simulink model "StateFlow_varB"  (R2022b)
settings: Solver=VariableStepAuto  StartTime=0.0  StopTime=500  FixedStep=0.001  RelTol=1e-3
InitFcn:
  | State_Flow_varB_setting
values from neighbouring files (symbols this model uses):
  Acceptable_press_offset = 5    [State_Flow_varB_setting.m]
  Desired_pressure_in_oxidiser_tank = 40    [State_Flow_varB_setting.m]
  Desired_pressure_in_pressure_section1 = 150    [State_Flow_varB_setting.m]
  Desired_pressure_in_pressure_section2 = 180    [State_Flow_varB_setting.m]
  s = struct    [State_Flow_varB_setting.m]
  Servo_open_limit = 20    [State_Flow_varB_setting.m]
  UDP_FC_send_packet_length = 68    [State_Flow_varB_setting.m]
  UDP_FC_send_sample_time = 0.05    [State_Flow_varB_setting.m]
  UDP_GSE_Curr_loop_receive_sample_time = 0.01    [State_Flow_varB_setting.m]
  UDP_GSE_IO_send_sample_time = 0.05    [State_Flow_varB_setting.m]
  UDP_GSE_send_packet_length = 68    [State_Flow_varB_setting.m]
libraries: simulink x36, slrealtimeiplib x16, slpidlib x6
(part 2 of 3)

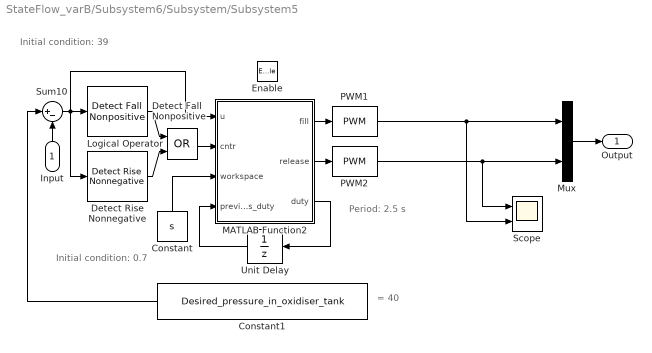
== system StateFlow_varB/Subsystem6/Subsystem/Subsystem5 ==
  note: Initial condition: 39
  note: Period: 2.5 s
  note: Initial condition: 0.7
  note: = 40
  Input : Inport
  Enable : EnablePort  StatesWhenEnabling=reset
  Constant : Constant  Value=s  OutDataTypeStr=Bus: s_bus
  Constant1 : Constant  Value=Desired_pressure_in_oxidiser_tank
  Detect Fall Nonpositive : simulink/Logic and Bit Operations/Detect Fall Nonpositive  vinit=Desired_pressure_in_oxidiser_tank-1  OutDataTypeStr=boolean
  Detect Rise Nonnegative : simulink/Logic and Bit Operations/Detect Rise Nonnegative  vinit=Desired_pressure_in_oxidiser_tank-1  OutDataTypeStr=boolean
  Logical Operator : Logic  Operator=OR  AllPortsSameDT=off  OutDataTypeStr=boolean
  MATLAB Function2 : MATLAB Function  TreatAsAtomicUnit=on
  Mux : Mux  Inputs=2
  PWM1 : simulink/Discontinuities/PWM  DisableCoverage=on  Period=2.5  InitialDelay=0  DisallowZeroDutyCycle=off  RunAtFixedTimeIntervals=off  SampleTime=0.1
  PWM2 : simulink/Discontinuities/PWM  DisableCoverage=on  Period=2.5  InitialDelay=0  DisallowZeroDutyCycle=off  RunAtFixedTimeIntervals=off  SampleTime=0.1
  Scope : Scope  NumInputPorts=2
  Sum10 : Sum  Inputs=|+-
  Unit Delay : UnitDelay  InitialCondition=0.7  SampleTime=-1  HasFrameUpgradeWarning=on
  Output : Outport
  wires:
  Logical Operator/1 -> MATLAB Function2/2(cntr)
  Detect Fall Nonpositive/1 -> Logical Operator/1
  Detect Rise Nonnegative/1 -> Logical Operator/2
  PWM2/1 -> Scope/1, Mux/2
  MATLAB Function2/2(release) -> PWM2/1
  MATLAB Function2/1(fill) -> PWM1/1
  PWM1/1 -> Scope/2, Mux/1
  Unit Delay/1 -> MATLAB Function2/4(previous_duty)
  MATLAB Function2/3(duty) -> Unit Delay/1
  Input/1 -> Sum10/2
  Mux/1 -> Output/1
  Constant/1 -> MATLAB Function2/3(workspace)
  Sum10/1 -> Detect Fall Nonpositive/1, MATLAB Function2/1(u), Detect Rise Nonnegative/1
  Constant1/1 -> Sum10/1

== system StateFlow_varB/Subsystem6/Subsystem/Subsystem6 ==
  Input : Inport
  Enable : EnablePort
  Constant : Constant  Value=Desired_pressure_in_oxidiser_tank
  Dead Zone2 : DeadZone  LowerValue=-Acceptable_press_offset  UpperValue=Acceptable_press_offset
  Gain3 : Gain  Gain=-1
  Mux : Mux  Inputs=2
  Relay3 : Relay  OnSwitchValue=Acceptable_press_offset  OffSwitchValue=0
  Relay4 : Relay  OnSwitchValue=Acceptable_press_offset  OffSwitchValue=0
  Sum7 : Sum  Inputs=|+-
  Output : Outport
  wires:
  Gain3/1 -> Relay4/1
  Relay4/1 -> Mux/2
  Dead Zone2/1 -> Relay3/1, Gain3/1
  Sum7/1 -> Dead Zone2/1
  Relay3/1 -> Mux/1
  Constant/1 -> Sum7/1
  Input/1 -> Sum7/2
  Mux/1 -> Output/1

== system StateFlow_varB/Subsystem6/Subsystem/Subsystem7 ==
  Input : Inport
  Enable : EnablePort
  Constant : Constant  Value=Desired_pressure_in_pressure_section2
  Dead Zone1 : DeadZone  LowerValue=-Acceptable_press_offset  UpperValue=Acceptable_press_offset  SaturateOnIntegerOverflow=off
  Gain2 : Gain  Gain=-1
  Mux : Mux  Inputs=2
  Relay1 : Relay  OnSwitchValue=Acceptable_press_offset  OffSwitchValue=0
  Relay2 : Relay  OnSwitchValue=Acceptable_press_offset  OffSwitchValue=0
  Sum5 : Sum  Inputs=|+-
  Output : Outport
  wires:
  Sum5/1 -> Dead Zone1/1
  Relay1/1 -> Mux/1
  Dead Zone1/1 -> Relay1/1, Gain2/1
  Gain2/1 -> Relay2/1
  Constant/1 -> Sum5/1
  Relay2/1 -> Mux/2
  Input/1 -> Sum5/2
  Mux/1 -> Output/1

== system StateFlow_varB/Subsystem6/Subsystem/Subsystem8 ==
  note: Period: 2 s
  note: Proportional (P): 0.008
  note: Saturation - Upper limit: 1
  note: Saturation - Lower limit: -1
  note: = 180
  Input : Inport
  Enable : EnablePort  StatesWhenEnabling=reset
  Constant : Constant  Value=Desired_pressure_in_pressure_section2
  Gain6 : Gain  Gain=-1
  Mux : Mux  Inputs=2
  PID Controller4 : slpidlib/PID Controller  Controller=P  Form=Parallel  TimeDomain=Discrete-time  UseExternalTs=off  SampleTime=-1  IntegratorMethod=Forward Euler  FilterMethod=Forward Euler  ControllerParametersSource=internal  P=0.008  I=0.01  UseKiTs=off  D=0  N=100  UseFilter=on  TunerSelectOption=Transfer Function Based (PID Tuner App)  InitialConditionSource=internal  InitialConditionForIntegrator=0  InitialConditionForFilter=0  DifferentiatorICPrevScaledInput=0  ExternalReset=none  TrackingMode=off  Kt=1  LimitOutput=on  SatLimitsSource=internal  UpperSaturationLimit=1  LowerSaturationLimit=-1  LinearizeAsGain=on  AntiWindupMode=none  Kb=1  LimitIntegrator=on  UpperIntegratorSaturationLimit=150  LowerIntegratorSaturationLimit=-inf  POutMin=[]  POutMax=[]  IOutMin=[]  IOutMax=[]  DOutMin=[]  DOutMax=[]  NOutMin=[]  NOutMax=[]  SumOutMin=[]  SumOutMax=[]  SaturationOutMin=[]  SaturationOutMax=[]  PParamMin=[]  PParamMax=[]  IParamMin=[]  IParamMax=[]  DParamMin=[]  DParamMax=[]  NParamMin=[]  NParamMax=[]  KbParamMin=[]  KbParamMax=[]  KtParamMin=[]  KtParamMax=[]  KbOutMin=[]  KbOutMax=[]  KtOutMin=[]  KtOutMax=[]  IntegratorOutMin=[]  IntegratorOutMax=[]  FilterOutMin=[]  FilterOutMax=[]  SumI1OutMin=[]  SumI1OutMax=[]  SumI2OutMin=[]  SumI2OutMax=[]  SumI3OutMin=[]  SumI3OutMax=[]  SumI4OutMin=[]  SumI4OutMax=[]  SumDOutMin=[]  SumDOutMax=[]  DifferentiatorOutMin=[]  DifferentiatorOutMax=[]  FilterDiffOutCoefMin=[]  FilterDiffOutCoefMax=[]  ReciprocalOutMin=[]  ReciprocalOutMax=[]  SumDenOutMin=[]  SumDenOutMax=[]  SumNumOutMin=[]  SumNumOutMax=[]  DivideOutMin=[]  DivideOutMax=[]  UdiffTsProdOutMin=[]  UdiffTsProdOutMax=[]  NTsProdOutMin=[]  NTsProdOutMax=[]  UintegralTsProdOutMin=[]  UintegralTsProdOutMax=[]  UngainTsProdOutMin=[]  UngainTsProdOutMax=[]  ClampingZeroOutDataTypeStr=Inherit: Inherit via back propagation  ClampingZeroOutMin=[]  ClampingZeroOutMax=[]  FilterDenConstantOutDataTypeStr=Inherit: Inherit via back propagation  FilterDenConstantOutMin=[]  FilterDenConstantOutMax=[]  PCopyOutDataTypeStr=Inherit: Inherit via back propagation  PCopyOutMin=[]  PCopyOutMax=[]  NCopyOutDataTypeStr=Inherit: Inherit via back propagation  NCopyOutMin=[]  NCopyOutMax=[]  IntegratorContinuousStateAttributes=''  IntegratorStateMustResolveToSignalObject=off  IntegratorRTWStateStorageClass=Auto  FilterContinuousStateAttributes=''  FilterStateMustResolveToSignalObject=off  FilterRTWStateStorageClass=Auto  ParallelPVariant=InternalParameters  IdealPVariant=Disabled  IVariant=Disabled  DVariant=Disabled  IntegratorVariant=Disabled  SatVariant=Enabled  AWVariant=Disabled  PCopyVariant=Disabled  TRVariant=Disabled  FdbkBlocksVariant=Forward  IdealPFdbkVariant=Disabled  SatFdbkVariant=Disabled  DerivativeFilterVariant=Disabled  NVariant=Disabled  NCopyVariant=Disabled_SignalSpec  FilterICVariant=Disabled  IntegratorICVariant=Disabled  ExternalResetVariant=Disabled  TRSumVariant=Passthrough  SumFdbkVariant=Disabled  SumVariant=Passthrough_P  TsampFilterVariant=InternalTs  TsampNgainVariant=Passthrough  TsampIntegralVariant=Disabled_SignalSpec  ExternalSaturationOutDataTypeStr=Inherit: Same as second input
  PWM12 : simulink/Discontinuities/PWM  DisableCoverage=on  Period=2  InitialDelay=0  DisallowZeroDutyCycle=off  RunAtFixedTimeIntervals=off  SampleTime=0.1
  PWM6 : simulink/Discontinuities/PWM  DisableCoverage=on  Period=2  InitialDelay=0  DisallowZeroDutyCycle=off  RunAtFixedTimeIntervals=off  SampleTime=0.1
  Scope : Scope  NumInputPorts=3
  Sum4 : Sum  Inputs=|+-
  Output : Outport
  wires:
  PID Controller4/1 -> PWM6/1, Scope/3, Gain6/1
  Gain6/1 -> PWM12/1
  Mux/1 -> Output/1
  PWM6/1 -> Scope/2, Mux/1
  PWM12/1 -> Scope/1, Mux/2
  Constant/1 -> Sum4/1
  Input/1 -> Sum4/2
  Sum4/1 -> PID Controller4/1

== system StateFlow_varB/Subsystem6/Subsystem/Subsystem9 ==
  note: Initial condition: 149
  note: Period: 2.5 s
  note: Initial condition: 0.2
  note: = 150
  Input : Inport
  Enable : EnablePort  StatesWhenEnabling=reset
  Constant : Constant  Value=s  OutDataTypeStr=Bus: s_bus
  Constant1 : Constant  Value=Desired_pressure_in_pressure_section1
  Detect Fall Nonpositive : simulink/Logic and Bit Operations/Detect Fall Nonpositive  vinit=Desired_pressure_in_pressure_section1-1  OutDataTypeStr=boolean
  Detect Rise Nonnegative : simulink/Logic and Bit Operations/Detect Rise Nonnegative  vinit=Desired_pressure_in_pressure_section1-1  OutDataTypeStr=boolean
  Logical Operator : Logic  Operator=OR  AllPortsSameDT=off  OutDataTypeStr=boolean
  MATLAB Function2 : MATLAB Function  TreatAsAtomicUnit=on
  Mux : Mux  Inputs=2
  PWM1 : simulink/Discontinuities/PWM  DisableCoverage=on  Period=2.5  InitialDelay=0  DisallowZeroDutyCycle=off  RunAtFixedTimeIntervals=off  SampleTime=0.1
  PWM2 : simulink/Discontinuities/PWM  DisableCoverage=on  Period=2.5  InitialDelay=0  DisallowZeroDutyCycle=off  RunAtFixedTimeIntervals=off  SampleTime=0.1
  Scope : Scope  NumInputPorts=2
  Sum10 : Sum  Inputs=|+-
  Unit Delay : UnitDelay  InitialCondition=0.2  SampleTime=-1  HasFrameUpgradeWarning=on
  Output : Outport
  wires:
  Logical Operator/1 -> MATLAB Function2/2(cntr)
  Detect Fall Nonpositive/1 -> Logical Operator/1
  Detect Rise Nonnegative/1 -> Logical Operator/2
  PWM2/1 -> Scope/1, Mux/2
  MATLAB Function2/2(release) -> PWM2/1
  MATLAB Function2/1(fill) -> PWM1/1
  PWM1/1 -> Scope/2, Mux/1
  Unit Delay/1 -> MATLAB Function2/4(previous_duty)
  MATLAB Function2/3(duty) -> Unit Delay/1
  Input/1 -> Sum10/2
  Mux/1 -> Output/1
  Constant/1 -> MATLAB Function2/3(workspace)
  Sum10/1 -> Detect Fall Nonpositive/1, MATLAB Function2/1(u), Detect Rise Nonnegative/1
  Constant1/1 -> Sum10/1

== system StateFlow_varB/Subsystem6/Subsystem3/Subsystem1 ==
  data_prev : Inport
  Constant : Constant  Value=s  OutDataTypeStr=Bus: s_bus
  Display : Display
  Display1 : Display
  MATLAB Function1 : MATLAB Function  TreatAsAtomicUnit=on
  UDP Receive : slrealtimeiplib/UDP Receive  useHostTargetConn=off  ipAddress=UDP_GSE_receive_local_IP  localPort=UDP_GSE_receive_local_PORT  rcvWidth=UDP_GSE_receive_receive_width  rcvFmAny=on  fmAddress='10.10.10.10'  sampleTime=UDP_GSE_Curr_loop_receive_sample_time/4  enableMessage=off  maxPackets=1
  y : Outport
  wires:
  UDP Receive/2 -> Display/1
  data_prev/1 -> MATLAB Function1/2(data_prev)
  MATLAB Function1/1(y) -> y/1
  Constant/1 -> MATLAB Function1/3(workspace)
  UDP Receive/1 -> Display1/1, MATLAB Function1/1(data_new)

== system StateFlow_varB/Subsystem6/Subsystem/Subsystem2/Subsystem1 ==
  Input : Inport
  Enable : EnablePort  StatesWhenEnabling=reset
  Constant : Constant  Value=UDP_GSE_send_packet_length
  Constant2 : Constant  Value=s  OutDataTypeStr=Bus: s_bus
  Constant5 : Constant  Value=s  OutDataTypeStr=Bus: s_bus
  Demux : Demux  Outputs=2
  MATLAB Function : MATLAB Function  TreatAsAtomicUnit=on
  MATLAB Function1 : MATLAB Function  TreatAsAtomicUnit=on
  Scope : Scope
  Scope1 : Scope
  UDP Send : slrealtimeiplib/UDP Send  useHostTargetConn=off  toAddress=UDP_GSE_send_to_IP  toPort=IO_card_2_port  sampleTime=UDP_GSE_IO_send_sample_time  enableMessage=off
  UDP Send1 : slrealtimeiplib/UDP Send  useHostTargetConn=off  toAddress=UDP_GSE_send_to_IP  toPort=IO_card_3_port  sampleTime=UDP_GSE_IO_send_sample_time  enableMessage=off
  wires:
  Input/1 -> Demux/1
  Constant5/1 -> MATLAB Function/2(workspace)
  Demux/1 -> Scope/1, MATLAB Function/1(input)
  Constant2/1 -> MATLAB Function1/2(workspace)
  Demux/2 -> Scope1/1, MATLAB Function1/1(input)
  MATLAB Function/1(code) -> UDP Send/1
  MATLAB Function1/1(code) -> UDP Send1/1
  Constant/1 -> UDP Send/2, UDP Send1/2

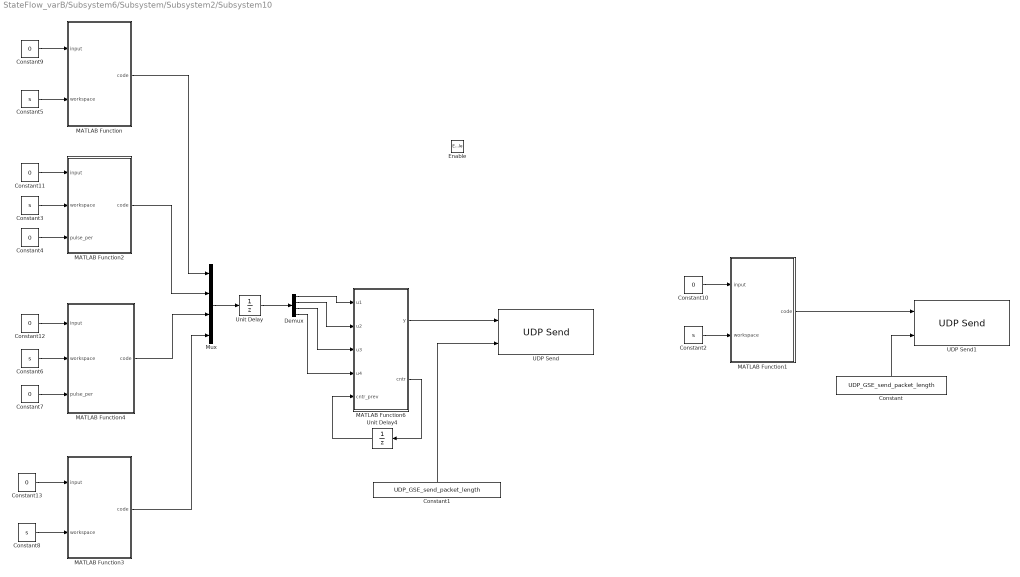
== system StateFlow_varB/Subsystem6/Subsystem/Subsystem2/Subsystem10 ==
  Enable : EnablePort  StatesWhenEnabling=reset
  Constant : Constant  Value=UDP_GSE_send_packet_length
  Constant1 : Constant  Value=UDP_GSE_send_packet_length
  Constant{4,7,9..13} (7 alike) : Constant  Value=0
  Constant{2..3,5..6,8} (5 alike) : Constant  Value=s  OutDataTypeStr=Bus: s_bus
  Demux : Demux
  MATLAB Function : MATLAB Function  TreatAsAtomicUnit=on
  MATLAB Function1 : MATLAB Function  TreatAsAtomicUnit=on
  MATLAB Function2 : MATLAB Function  TreatAsAtomicUnit=on
  MATLAB Function3 : MATLAB Function  TreatAsAtomicUnit=on
  MATLAB Function4 : MATLAB Function  TreatAsAtomicUnit=on
  MATLAB Function6 : MATLAB Function  TreatAsAtomicUnit=on
  Mux : Mux
  UDP Send : slrealtimeiplib/UDP Send  useHostTargetConn=off  toAddress=UDP_GSE_send_to_IP  toPort=IO_card_2_port  sampleTime=UDP_GSE_IO_send_sample_time  enableMessage=off
  UDP Send1 : slrealtimeiplib/UDP Send  useHostTargetConn=off  toAddress=UDP_GSE_send_to_IP  toPort=IO_card_3_port  sampleTime=UDP_GSE_IO_send_sample_time  enableMessage=off
  Unit Delay : UnitDelay  SampleTime=UDP_GSE_IO_send_sample_time*4  HasFrameUpgradeWarning=on
  Unit Delay4 : UnitDelay  InitialCondition=1  SampleTime=UDP_GSE_IO_send_sample_time  HasFrameUpgradeWarning=on
  wires:
  Constant2/1 -> MATLAB Function1/2(workspace)
  MATLAB Function1/1(code) -> UDP Send1/1
  Constant10/1 -> MATLAB Function1/1(input)
  Constant/1 -> UDP Send1/2
  MATLAB Function6/1(y) -> UDP Send/1
  MATLAB Function2/1(code) -> Mux/2
  MATLAB Function4/1(code) -> Mux/3
  MATLAB Function3/1(code) -> Mux/4
  Mux/1 -> Unit Delay/1
  Constant8/1 -> MATLAB Function3/2(workspace)
  Constant12/1 -> MATLAB Function4/1(input)
  Constant6/1 -> MATLAB Function4/2(workspace)
  Constant5/1 -> MATLAB Function/2(workspace)
  Constant4/1 -> MATLAB Function2/3(pulse_per)
  MATLAB Function/1(code) -> Mux/1
  Constant7/1 -> MATLAB Function4/3(pulse_per)
  Constant13/1 -> MATLAB Function3/1(input)
  Constant9/1 -> MATLAB Function/1(input)
  Constant3/1 -> MATLAB Function2/2(workspace)
  Constant11/1 -> MATLAB Function2/1(input)
  Unit Delay/1 -> Demux/1
  Demux/1 -> MATLAB Function6/1(u1)
  Demux/2 -> MATLAB Function6/2(u2)
  Demux/3 -> MATLAB Function6/3(u3)
  Demux/4 -> MATLAB Function6/4(u4)
  MATLAB Function6/2(cntr) -> Unit Delay4/1
  Unit Delay4/1 -> MATLAB Function6/5(cntr_prev)
  Constant1/1 -> UDP Send/2

== system StateFlow_varB/Subsystem6/Subsystem/Subsystem2/Subsystem11 ==
  In1 : Inport
  In2 : Inport  Port=2
  Enable : EnablePort
  UDP Send5 : slrealtimeiplib/UDP Send  useHostTargetConn=off  toAddress=UDP_GSE_send_to_IP  toPort=UDP_GSE_send_to_PORT  sampleTime=UDP_GSE_IO_send_sample_time  enableMessage=off
  wires:
  In2/1 -> UDP Send5/2
  In1/1 -> UDP Send5/1

== system StateFlow_varB/Subsystem6/Subsystem/Subsystem2/Subsystem5 ==
  note: To port: 10003
  note: To IP address: 127.0.0.1
  note: Sample time: 0.05
  note: To port: 10004
  note: To IP address: 127.0.0.1
  note: Sample time: 0.05
  Input : Inport
  Enable : EnablePort  StatesWhenEnabling=reset
  Constant : Constant  Value=UDP_GSE_send_packet_length
  Constant2 : Constant  Value=s  OutDataTypeStr=Bus: s_bus
  Constant5 : Constant  Value=s  OutDataTypeStr=Bus: s_bus
  Demux : Demux  Outputs=2
  MATLAB Function : MATLAB Function  TreatAsAtomicUnit=on
  MATLAB Function1 : MATLAB Function  TreatAsAtomicUnit=on
  UDP Send : slrealtimeiplib/UDP Send  useHostTargetConn=off  toAddress=UDP_GSE_send_to_IP  toPort=IO_card_2_port  sampleTime=UDP_GSE_IO_send_sample_time  enableMessage=off
  UDP Send1 : slrealtimeiplib/UDP Send  useHostTargetConn=off  toAddress=UDP_GSE_send_to_IP  toPort=IO_card_3_port  sampleTime=UDP_GSE_IO_send_sample_time  enableMessage=off
  wires:
  Input/1 -> Demux/1
  Constant5/1 -> MATLAB Function/2(workspace)
  Demux/1 -> MATLAB Function/1(input)
  Constant2/1 -> MATLAB Function1/2(workspace)
  Demux/2 -> MATLAB Function1/1(input)
  MATLAB Function/1(code) -> UDP Send/1
  MATLAB Function1/1(code) -> UDP Send1/1
  Constant/1 -> UDP Send/2, UDP Send1/2

== system StateFlow_varB/Subsystem6/Subsystem/Subsystem2/Subsystem6 ==
  In1 : Inport
  Enable : EnablePort  StatesWhenEnabling=reset
  Constant1 : Constant  Value=UDP_FC_send_packet_length
  Constant3 : Constant  Value=s  OutDataTypeStr=Bus: s_bus
  Constant6 : Constant  Value=s  OutDataTypeStr=Bus: s_bus
  Demux : Demux
  Demux1 : Demux  Outputs=2
  MATLAB Function2 : MATLAB Function  TreatAsAtomicUnit=on
  MATLAB Function4 : MATLAB Function  TreatAsAtomicUnit=on
  MATLAB Function6 : MATLAB Function  TreatAsAtomicUnit=on
  Mux : Mux  Inputs=2
  UDP Send2 : slrealtimeiplib/UDP Send  useHostTargetConn=off  toAddress=UDP_FC_send_to_IP  toPort=IO_card_2_port  sampleTime=UDP_GSE_IO_send_sample_time  enableMessage=off
  Unit Delay2 : UnitDelay  SampleTime=UDP_FC_send_sample_time*2  HasFrameUpgradeWarning=on
  Unit Delay4 : UnitDelay  InitialCondition=1  SampleTime=UDP_FC_send_sample_time  HasFrameUpgradeWarning=on
  wires:
  In1/1 -> Demux/1
  Constant3/1 -> MATLAB Function2/2(workspace)
  Demux/1 -> MATLAB Function2/1(input)
  Constant6/1 -> MATLAB Function4/2(workspace)
  Constant1/1 -> UDP Send2/2
  Demux/4 -> MATLAB Function4/3(pulse_per)
  Demux/2 -> MATLAB Function4/1(input)
  Demux/3 -> MATLAB Function2/3(pulse_per)
  MATLAB Function2/1(code) -> Mux/1
  MATLAB Function4/1(code) -> Mux/2
  Mux/1 -> Unit Delay2/1
  Unit Delay2/1 -> Demux1/1
  MATLAB Function6/2(cntr) -> Unit Delay4/1
  Unit Delay4/1 -> MATLAB Function6/3(cntr_prev)
  Demux1/1 -> MATLAB Function6/1(u1)
  Demux1/2 -> MATLAB Function6/2(u2)
  MATLAB Function6/1(y) -> UDP Send2/1

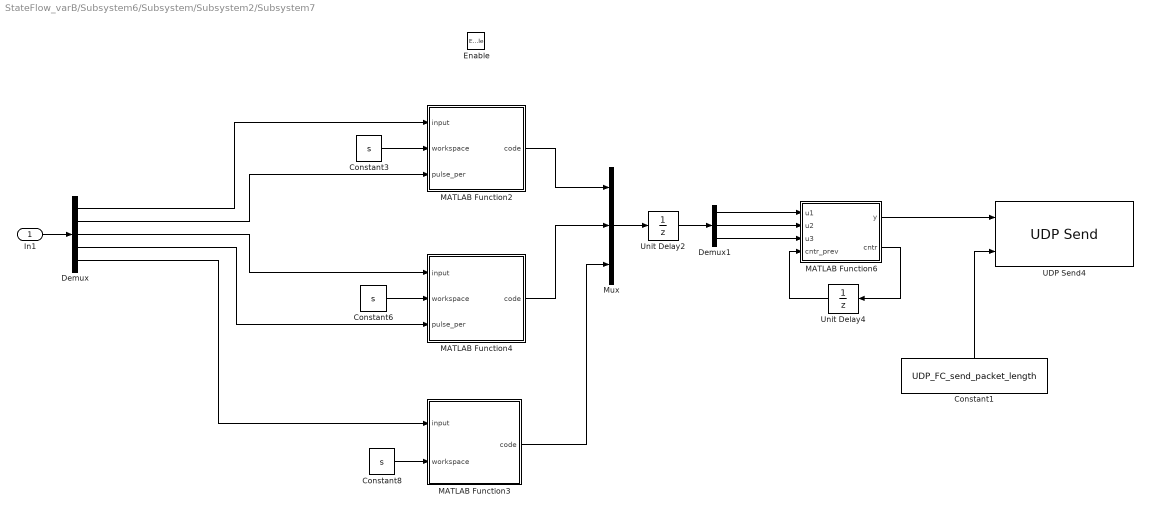
== system StateFlow_varB/Subsystem6/Subsystem/Subsystem2/Subsystem7 ==
  In1 : Inport
  Enable : EnablePort  StatesWhenEnabling=reset
  Constant1 : Constant  Value=UDP_FC_send_packet_length
  Constant3 : Constant  Value=s  OutDataTypeStr=Bus: s_bus
  Constant6 : Constant  Value=s  OutDataTypeStr=Bus: s_bus
  Constant8 : Constant  Value=s  OutDataTypeStr=Bus: s_bus
  Demux : Demux  Outputs=5
  Demux1 : Demux  Outputs=3
  MATLAB Function2 : MATLAB Function  TreatAsAtomicUnit=on
  MATLAB Function3 : MATLAB Function  TreatAsAtomicUnit=on
  MATLAB Function4 : MATLAB Function  TreatAsAtomicUnit=on
  MATLAB Function6 : MATLAB Function  TreatAsAtomicUnit=on
  Mux : Mux  Inputs=3
  UDP Send4 : slrealtimeiplib/UDP Send  useHostTargetConn=off  toAddress=UDP_FC_send_to_IP  toPort=IO_card_2_port  sampleTime=UDP_GSE_IO_send_sample_time  enableMessage=off
  Unit Delay2 : UnitDelay  SampleTime=UDP_GSE_IO_send_sample_time*3  HasFrameUpgradeWarning=on
  Unit Delay4 : UnitDelay  InitialCondition=1  SampleTime=UDP_GSE_IO_send_sample_time  HasFrameUpgradeWarning=on
  wires:
  Constant3/1 -> MATLAB Function2/2(workspace)
  Constant6/1 -> MATLAB Function4/2(workspace)
  Constant1/1 -> UDP Send4/2
  In1/1 -> Demux/1
  Demux/1 -> MATLAB Function2/1(input)
  Demux/4 -> MATLAB Function4/3(pulse_per)
  Demux/2 -> MATLAB Function2/3(pulse_per)
  Demux/3 -> MATLAB Function4/1(input)
  MATLAB Function2/1(code) -> Mux/1
  MATLAB Function4/1(code) -> Mux/2
  Mux/1 -> Unit Delay2/1
  MATLAB Function6/2(cntr) -> Unit Delay4/1
  Demux1/1 -> MATLAB Function6/1(u1)
  Unit Delay4/1 -> MATLAB Function6/4(cntr_prev)
  Demux1/2 -> MATLAB Function6/2(u2)
  Unit Delay2/1 -> Demux1/1
  MATLAB Function6/1(y) -> UDP Send4/1
  Constant8/1 -> MATLAB Function3/2(workspace)
  Demux/5 -> MATLAB Function3/1(input)
  MATLAB Function3/1(code) -> Mux/3
  Demux1/3 -> MATLAB Function6/3(u3)

== system StateFlow_varB/Subsystem6/Subsystem/Subsystem2/Subsystem8 ==
  Input : Inport
  Enable : EnablePort
  Constant : Constant  Value=UDP_GSE_send_packet_length
  Constant8 : Constant  Value=s  OutDataTypeStr=Bus: s_bus
  MATLAB Function3 : MATLAB Function  TreatAsAtomicUnit=on
  UDP Send3 : slrealtimeiplib/UDP Send  useHostTargetConn=off  toAddress=UDP_GSE_send_to_IP  toPort=IO_card_2_port  sampleTime=UDP_GSE_IO_send_sample_time  enableMessage=off
  wires:
  Constant8/1 -> MATLAB Function3/2(workspace)
  Input/1 -> MATLAB Function3/1(input)
  MATLAB Function3/1(code) -> UDP Send3/1
  Constant/1 -> UDP Send3/2

== system StateFlow_varB/Subsystem6/Subsystem/Subsystem2/Subsystem9 ==
  Input : Inport
  Enable : EnablePort  StatesWhenEnabling=reset
  Constant : Constant  Value=UDP_GSE_send_packet_length
  Constant6 : Constant  Value=s  OutDataTypeStr=Bus: s_bus
  Constant8 : Constant  Value=s  OutDataTypeStr=Bus: s_bus
  Demux : Demux  Outputs=3
  Demux1 : Demux  Outputs=2
  MATLAB Function3 : MATLAB Function  TreatAsAtomicUnit=on
  MATLAB Function4 : MATLAB Function  TreatAsAtomicUnit=on
  MATLAB Function6 : MATLAB Function  TreatAsAtomicUnit=on
  Mux : Mux  Inputs=2
  UDP Send4 : slrealtimeiplib/UDP Send  useHostTargetConn=off  toAddress=UDP_FC_send_to_IP  toPort=IO_card_2_port  sampleTime=UDP_GSE_IO_send_sample_time  enableMessage=off
  Unit Delay2 : UnitDelay  SampleTime=UDP_GSE_IO_send_sample_time*2  HasFrameUpgradeWarning=on
  Unit Delay4 : UnitDelay  InitialCondition=1  SampleTime=UDP_GSE_IO_send_sample_time  HasFrameUpgradeWarning=on
  wires:
  Constant6/1 -> MATLAB Function4/2(workspace)
  Constant/1 -> MATLAB Function6/3(length), UDP Send4/2
  Constant8/1 -> MATLAB Function3/2(workspace)
  Demux/1 -> MATLAB Function4/1(input)
  Demux/2 -> MATLAB Function4/3(pulse_per)
  Demux/3 -> MATLAB Function3/1(input)
  Input/1 -> Demux/1
  MATLAB Function4/1(code) -> Mux/1
  MATLAB Function3/1(code) -> Mux/2
  Mux/1 -> Unit Delay2/1
  MATLAB Function6/2(cntr) -> Unit Delay4/1
  Demux1/1 -> MATLAB Function6/1(u1)
  Unit Delay4/1 -> MATLAB Function6/4(cntr_prev)
  Demux1/2 -> MATLAB Function6/2(u2)
  Unit Delay2/1 -> Demux1/1
  MATLAB Function6/1(y) -> UDP Send4/1

== matlab function StateFlow_varB/Subsystem6/Subsystem/Subsystem2/Subsystem1/MATLAB Function ==
  data: input input; code output; workspace input
function code = fcn(input, workspace)

if input == 1
    code = workspace.N2_fill_valve_open; 
else 
    code = workspace.N2_fill_valve_close; 
end
     
end

== matlab function StateFlow_varB/Subsystem6/Subsystem/Subsystem2/Subsystem1/MATLAB Function1 ==
  data: input input; code output; workspace input
function code = fcn(input, workspace)

if input == 1
    code = workspace.N2_release_valve_open;
else
    code = workspace.N2_release_valve_close;
end
     
end

== stateflow chart StateFlow_varB/Subsystem6/Subsystem/Chart ==
  state Pressure_section_pressurization
    entry:
    Pressure_section_pressurization = 1;
    Pressure_section_cntr = 0;
    state Pressure_section_pressurization_Phase_1
      Pressure_section_pressurization_Phase_1 -> (junction 67) [order 1]
      (junction 67) -> (junction 68) [order 1] : [abs(Pressure_section_pressure - Pressure_section_pressure_des) > Acc_Press_Offset]
      (junction 67) -> (junction 69) [order 2]
      (junction 68) -> (junction 70) : {Pressure_section_cntr = 0;}
      (junction 70) -> (junction 69)
      (junction 69) -> (junction 71)
    state Pressure_section_pressurization_Phase_2
      entry:
      Pressure_section_cntr = Pressure_section_cntr + 1
    state Pressure_section_pressurization_Exit_state
      entry:
      Pressure_section_pressurization = 0;
    (default) -> Pressure_section_pressurization_Phase_1
    Pressure_section_pressurization_Phase_1 -> Pressure_section_pressurization_Phase_2 [order 1] : [abs(Pressure_section_pressure - Pressure_section_pressure_des) < Acc_Press_Offset]
    Pressure_section_pressurization_Phase_2 -> Pressure_section_pressurization_Phase_1 [order 2] : [after(Press_Transition_time_const, sec)]
    Pressure_section_pressurization_Phase_2 -> Pressure_section_pressurization_Exit_state [order 1] : [Pressure_section_cntr == Num_dec_time_cycles]
  state Pressure_venting
    entry:
    Pressure_venting = 1;
    Pressure_venting_cntr = 0;
    state Pressure_venting_Phase_1
      Pressure_venting_Phase_1 -> (junction 87) [order 1]
      (junction 87) -> (junction 89) [order 1] : [abs(Oxidiser_tank_pressure - Oxidiser_tank_pressure_des) > Acc_Press_Offset]
      (junction 87) -> (junction 90) [order 2]
      (junction 89) -> (junction 94) : {Pressure_venting_cntr = 0;}
      (junction 94) -> (junction 90)
      (junction 90) -> (junction 92)
    state Pressure_venting_Phase_2
      entry:
      Pressure_venting_cntr = Pressure_venting_cntr + 1;
    state Pressure_venting_Exit_state
      entry:
      Pressure_venting = 0;
    (default) -> Pressure_venting_Phase_1
    Pressure_venting_Phase_1 -> Pressure_venting_Phase_2 [order 1] : [abs(Oxidiser_tank_pressure - Oxidiser_tank_pressure_des) < Acc_Press_Offset]
    Pressure_venting_Phase_2 -> Pressure_venting_Phase_1 [order 2] : [after(Press_Transition_time_const, sec)]
    Pressure_venting_Phase_2 -> Pressure_venting_Exit_state [order 1] : [Pressure_venting_cntr == Num_dec_time_cycles]
  state Oxidiser_fueling_pre_phase
    entry:
    Oxidiser_fueling_pre_phase_cntrl = 1;
    Venting_valve = 0;
    Releasing_valve = 1;
    Oxidiser_fueling_valve = 1;
    state Oxidiser_fueling_pre_phase_init
    state Oxidiser_fueling_exit_state
    (default) -> Oxidiser_fueling_pre_phase_init
    Oxidiser_fueling_pre_phase_init -> Oxidiser_fueling_exit_state : [High_servo_state == 0 && Low_servo_state == 90 && N2O_Fill_valve_state == 0]
  state Oxidiser_fueling
    entry:
    Oxidiser_fueling_cntrl = 1;
    state Oxidiser_fueling_valve_open2
      entry:
      Oxidiser_fueling_valve = 1;
    (default) -> Oxidiser_fueling_valve_open2
  state Oxidiser_fueling_post_phase
    entry:
    Oxidiser_fueling_post_phase_cntrl = 1;
    Oxidiser_fueling_valve = 0;
    Releasing_valve = 0;
    state Oxidiser_fueling_post_phase_init
    state Oxidiser_fueling_post_state
    (default) -> Oxidiser_fueling_post_phase_init
    Oxidiser_fueling_post_phase_init -> Oxidiser_fueling_post_state : [ Low_servo_state == 0 && N2O_Fill_valve_state == 255]
  state Pressure_section_post_pressurization1
    entry:
    Pressure_section_post_pressurization = 1;
    Pressure_section_post_cntr = 0;
    state Pressure_section_post_pressurization_Phase_1
      Pressure_section_post_pressurization_Phase_1 -> (junction 153) [order 1]
      (junction 153) -> (junction 161) [order 1] : [abs(Pressure_section_pressure - Pressure_section_post_pressure_des) > Acc_Press_Offset]
      (junction 153) -> (junction 168) [order 2]
      (junction 161) -> (junction 165) : {Pressure_section_post_cntr = 0;}
      (junction 165) -> (junction 168)
      (junction 168) -> (junction 169)
    state Pressure_section_post_pressurization_Phase_2
      entry:
      Pressure_section_post_cntr = Pressure_section_post_cntr + 1
    state Pressure_section_post_pressurization_Exit_state
      entry:
      Pressure_section_post_pressurization = 0;
    (default) -> Pressure_section_post_pressurization_Phase_1
    Pressure_section_post_pressurization_Phase_2 -> Pressure_section_post_pressurization_Phase_1 [order 2] : [after(Press_Transition_time_const, sec)]
    Pressure_section_post_pressurization_Phase_1 -> Pressure_section_post_pressurization_Phase_2 [order 1] : [abs(Pressure_section_pressure - Pressure_section_post_pressure_des) < Acc_Press_Offset]
    Pressure_section_post_pressurization_Phase_2 -> Pressure_section_post_pressurization_Exit_state [order 1] : [Pressure_section_post_cntr == Num_dec_time_cycles]
  state END_phase
    entry:
    END_Phase_cntrl = 1;
    Releasing_valve = 0;
    Venting_valve = 0;
    Oxidiser_fueling_valve = 0;
  (default) -> Pressure_section_pressurization
  Pressure_section_pressurization_Exit_state -> Pressure_venting : [after(State_transition_time_const,sec)]
  Pressure_venting_Exit_state -> Oxidiser_fueling_pre_phase : [after(State_transition_time_const,sec)]
  Oxidiser_fueling_exit_state -> Oxidiser_fueling : [after(State_transition_time_const,sec)]{Oxidiser_fueling_pre_phase_cntrl = 0;}
  Oxidiser_fueling_valve_open2 -> Oxidiser_fueling_post_phase : [Oxidiser_fueling_valve_time_open == Oxidiser_fueling_exit && Oxidiser_fueling_valve_cntrl_sig == 1 ]{Oxidiser_fueling_cntrl  = 0;}
  Oxidiser_fueling_post_state -> Pressure_section_post_pressurization1 : [after(State_transition_time_const,sec)]{Oxidiser_fueling_post_phase_cntrl = 0;}
  Pressure_section_post_pressurization_Exit_state -> END_phase : [after(State_transition_time_const,sec)]
  data: Pressure_section_pressurization output; Pressure_section_pressure input =150; Pressure_venting output; Oxidiser_fueling_pre_phase_cntrl output; Acc_Press_Offset constant double =Acceptable_press_offset; Press_Transition_time_const constant double =Press_Transition_time_const; Pressure_section_pressure_des constant double =Desired_pressure_in_pressure_section1; Num_dec_time_cycles local =Number_of_decisive_time_cycles; Pressure_venting_cntr local =0; Oxidiser_tank_pressure_des constant double =Desired_pressure_in_oxidiser_tank; Oxidiser_tank_pressure input; State_transition_time_const constant double =Large_State_transition_time_const; Pressure_section_cntr local =0; Venting_valve output; Small_State_transition_time_const local =Small_State_transition_time_const; Oxidiser_fueling_exit constant double =Oxidiser_fueling_exit; Releasing_valve output; Oxidiser_fueling_cntrl output; Oxidiser_fueling_valve output; Oxidiser_fueling_post_phase_cntrl output; Pressure_section_post_cntr local =0; Pressure_section_post_pressure_des constant double =Desired_pressure_in_pressure_section2; END_Phase_cntrl output; Pressure_section_post_pressurization output; N2_Fill_valve_state input; N2_Release_valve_state input; N2O_Fill_valve_state input; N2O_Release_valve_state input; High_servo_state input; Low_servo_state input; Oxidiser_fueling_valve_time_open input; Oxidiser_fueling_valve_cntrl_sig input

== matlab function StateFlow_varB/Subsystem6/Subsystem3/MATLAB Function ==
  data: val_const input; valves_state input; workspace input; u input; y output
function y = fcn(val_const, valves_state, workspace, u)

coder.extrinsic('set_param')

if u >= val_const
    set_param('StateFlow_varB/Subsystem6/Subsystem3/Constant', 'Value', sprintf('%f',u))
    y = 0;
else
   first_valve = valves_state(1);
   second_valve = valves_state(2);
   if ~(first_valve || second_valve)
       if u <= (val_const - workspace.Pressure_drop_const)
           set_param('StateFlow_varB/Subsystem6/Constant', 'Value', '0')
           y = 1;
       else
           y = 0;
       end
   else
       set_param('StateFlow_varB/Subsystem6/Subsystem3/Constant', 'Value', sprintf('%f',u))
       y = 0;
   end
end

end

== matlab function StateFlow_varB/Subsystem6/Subsystem10/MATLAB Function ==
  data: input input; code output; workspace input
function code = fcn(input, workspace)

if input == 1
    code = workspace.N2_fill_valve_open;
else
    code = workspace.N2_fill_valve_close;
end
     
end

== matlab function StateFlow_varB/Subsystem6/Subsystem10/MATLAB Function1 ==
  data: input input; code output; workspace input
function code = fcn(input, workspace)

if input == 1
    code = workspace.N2_release_valve_open;
else
    code = workspace.N2_release_valve_close;
end
     
end

== matlab function StateFlow_varB/Subsystem6/Subsystem10/MATLAB Function2 ==
  data: input input; code output; workspace input; pulse_per input
function code = fcn(input, workspace, pulse_per)

coder.extrinsic('set_param')

if input == 1
    code = workspace.High_servo_open;
else
    code = workspace.High_servo_close;
end


% if pulse_per == 0
%     if input == 1
%         code = workspace.High_servo_open;
%     else
%         code = workspace.High_servo_close;
%     end
% else
%     %comment THIS section if servos are controlled via GSE
%     code = uint8([workspace.FC_ID, workspace.FC_PACKET_LENGTH, workspace.FC_GND_MSG_SERVO_CTRL, workspace.FC_SERVO_PULSE, workspace.FC_SERVO_IGNORE, typecast(uint32(pulse_per), 'uint8'), zeros(1,24)]);
%     set_param('StateFlow_varB/Subsystem6/Constant2', 'Value', '0') %pulse_per is in miliseconds
%     %counting with big endian format
% end

end

== matlab function StateFlow_varB/Subsystem6/Subsystem/Subsystem2/Subsystem5/MATLAB Function ==
  data: input input; code output; workspace input
function code = fcn(input, workspace)

if input == 1
    code = workspace.N2_fill_valve_open; 
else 
    code = workspace.N2_fill_valve_close; 
end
     
end

== matlab function StateFlow_varB/Subsystem6/Subsystem1/MATLAB Function6 ==
  data: u1 input; u2 input; u3 input; u4 input; y output; cntr_prev input; cntr output
function [y, cntr] = fcn(u1, u2, u3, u4, cntr_prev)


y = uint8(zeros(1,68));

switch cntr_prev
    case 1
        y = u1;
    case 2
        y = u2;
    case 3
        y = u3;
    case 4
        y = u4;
end

if cntr_prev < 4
    cntr = cntr_prev + 1;
else
    cntr = 1;
end

== matlab function StateFlow_varB/Subsystem6/Subsystem1/MATLAB Function7 ==
  data: u1 input; u2 input; y output; cntr_prev input; cntr output
function [y, cntr] = fcn(u1, u2, cntr_prev)


y = uint8(zeros(1,68));

switch cntr_prev
    case 1
        y = u1;
    case 2
        y = u2;
end

if cntr_prev < 2
    cntr = cntr_prev + 1;
else
    cntr = 1;
end

== matlab function StateFlow_varB/Subsystem6/Subsystem/Subsystem2/Subsystem5/MATLAB Function1 ==
  data: input input; code output; workspace input
function code = fcn(input, workspace)

if input == 1
    code = workspace.N2_release_valve_open;
else
    code = workspace.N2_release_valve_close;
end
     
end

== matlab function StateFlow_varB/Subsystem6/Subsystem/Subsystem2/Subsystem6/MATLAB Function2 ==
  data: input input; code output; workspace input; pulse_per input
function code = fcn(input, workspace, pulse_per)

coder.extrinsic('set_param')

if input == 1
    code = workspace.High_servo_open;
else
    code = workspace.High_servo_close;
end


% if pulse_per == 0
%     if input == 1
%         code = workspace.High_servo_open;
%     else
%         code = workspace.High_servo_close;
%     end
% else
%     %comment THIS section if servos are controlled via GSE
%     code = uint8([workspace.FC_ID, workspace.FC_PACKET_LENGTH, workspace.FC_GND_MSG_SERVO_CTRL, workspace.FC_SERVO_PULSE, workspace.FC_SERVO_IGNORE, typecast(uint32(pulse_per), 'uint8'), zeros(1,24)]);
%     set_param('StateFlow_varB/Subsystem6/Constant2', 'Value', '0') %pulse_per is in miliseconds
%     %counting with big endian format
% end

end

== matlab function StateFlow_varB/Subsystem6/Subsystem/Subsystem2/Subsystem6/MATLAB Function4 ==
  data: input input; code output; workspace input; pulse_per input
function code = fcn(input, workspace, pulse_per)

coder.extrinsic('set_param')

if input == 1
    code = workspace.Low_servo_open;
else
    code = workspace.Low_servo_close;
end

% if pulse_per == 0
%     if input == 1
%         code = workspace.Low_servo_open;
%     else
%         code = workspace.Low_servo_close;
%     end
% else
%     %comment THIS section if servos are controlled via GSE
%     code = uint8([workspace.FC_ID, workspace.FC_PACKET_LENGTH, workspace.FC_GND_MSG_SERVO_CTRL, workspace.FC_SERVO_PULSE, workspace.FC_SERVO_IGNORE, typecast(uint32(pulse_per), 'uint8'), zeros(1,24)]);
%     set_param('StateFlow_varB/Subsystem6/Constant3', 'Value', '0') %pulse_per is in miliseconds
%     %counting with big endian format
% end

end

== matlab function StateFlow_varB/Subsystem6/Subsystem/Subsystem2/Subsystem7/MATLAB Function2 ==
  data: input input; code output; workspace input; pulse_per input
function code = fcn(input, workspace, pulse_per)

coder.extrinsic('set_param')

if input == 1
    code = workspace.High_servo_open;
else
    code = workspace.High_servo_close;
end

% if pulse_per == 0
%     if input == 1
%         code = workspace.High_servo_open;
%     else
%         code = workspace.High_servo_close;
%     end
% else
%     %comment THIS section if servos are controlled via GSE
%     code = uint8([workspace.FC_ID, workspace.FC_PACKET_LENGTH, workspace.FC_GND_MSG_SERVO_CTRL, workspace.FC_SERVO_PULSE, workspace.FC_SERVO_IGNORE, typecast(uint32(pulse_per), 'uint8'), zeros(1,24)]);
%     set_param('StateFlow_varB/Subsystem6/Constant2', 'Value', '0') %pulse_per is in miliseconds
%     %counting with big endian format
% end

end

== matlab function StateFlow_varB/Subsystem6/Subsystem/Subsystem2/Subsystem7/MATLAB Function4 ==
  data: input input; code output; workspace input; pulse_per input
function code = fcn(input, workspace, pulse_per)

coder.extrinsic('set_param')

if input == 1
    code = workspace.Low_servo_open;
else
    code = workspace.Low_servo_close;
end

% if pulse_per == 0
%     if input == 1
%         code = workspace.Low_servo_open;
%     else
%         code = workspace.Low_servo_close;
%     end
% else
%     %comment THIS section if servos are controlled via GSE
%     code = uint8([workspace.FC_ID, workspace.FC_PACKET_LENGTH, workspace.FC_GND_MSG_SERVO_CTRL, workspace.FC_SERVO_IGNORE, workspace.FC_SERVO_PULSE, typecast(uint32(pulse_per), 'uint8'), zeros(1,24)]);
%     set_param('StateFlow_varB/Subsystem6/Constant3', 'Value', '0') %pulse_per is in miliseconds
%     %counting with big endian format
% end

end

== matlab function StateFlow_varB/Subsystem6/Subsystem/Subsystem2/Subsystem8/MATLAB Function3 ==
  data: input input; code output; workspace input
function code = fcn(input, workspace)

if input == 1
    code = workspace.N2O_fill_valve_open;
else
    code = workspace.N2O_fill_valve_close;
end

end

== matlab function StateFlow_varB/MATLAB Function ==
  data: u input; y output; inside input
function y  = fcn(u, inside)

a = inside.pokus;
y = a;

== matlab function StateFlow_varB/Subsystem6/Subsystem/Subsystem1/MATLAB Function ==
  data: u1 input; y output; u2 input; workspace input
function y = fcn(u1, u2, workspace)

coder.extrinsic('set_param')
set_param('StateFlow_varB/Subsystem6/Constant2', 'Value', u1*workspace.FC_PWM_period) %pulse_per is in miliseconds
set_param('StateFlow_varB/Subsystem6/Constant3', 'Value', u2*workspace.FC_PWM_period) %pulse_per is in miliseconds
%adjust UDP_FC_send_sample_time to larger value (for example 2s)

y = u1;

== matlab function StateFlow_varB/Subsystem6/Subsystem/Subsystem12/MATLAB Function2 ==
  data: u input; fill output; prev_u input; release output; workspace input; duty output; previous_duty input
function [fill, release, duty]= fcn(u, prev_u, workspace, previous_duty)

duty = previous_duty;
if u * prev_u < 0
    duty = previous_duty / 2;
end

if u > 5
    fill = duty;
    release = 0;
elseif u < -5
    release = duty;
    fill = 0;
else
    fill = 0;
    release = 0;
end

== matlab function StateFlow_varB/Subsystem6/Subsystem/Subsystem16/MATLAB Function2 ==
  data: u input; cntr input; fill output; release output; workspace input; duty output; previous_duty input
function [fill, release, duty]= fcn(u, ...
                                    cntr, ...
                                    workspace, ...
                                    previous_duty)

%Halving duty cycle
duty = previous_duty;
if cntr
    duty = previous_duty / 2;
end

%Deciding which valve should be open
if u > 5
    fill = duty;
    release = 0;
elseif u < -5
    release = duty;
    fill = 0;
else
    fill = 0;
    release = 0;
end

== matlab function StateFlow_varB/Subsystem6/Subsystem/Subsystem5/MATLAB Function2 ==
  data: u input; cntr input; fill output; release output; workspace input; duty output; previous_duty input
function [fill, release, duty]= fcn(u, ...
                                    cntr, ...
                                    workspace, ...
                                    previous_duty)

%Halving duty cycle
duty = previous_duty;
if cntr
    duty = previous_duty / 2;
end

%Deciding which valve should be open
if u > workspace.Acceptable_press_offset
    fill = duty;
    release = 0;
elseif u < -workspace.Acceptable_press_offset
    release = duty;
    fill = 0;
else
    fill = 0;
    release = 0;
end

== matlab function StateFlow_varB/Subsystem6/Subsystem/Subsystem14/MATLAB Function ==
  data: u1 input; y output; u2 input; workspace input
function y = fcn(u1, u2, workspace)

coder.extrinsic('set_param')
set_param('StateFlow_varB/Subsystem6/Constant2', 'Value', u1*workspace.FC_PWM_period) %pulse_per is in miliseconds
set_param('StateFlow_varB/Subsystem6/Constant3', 'Value', u2*workspace.FC_PWM_period) %pulse_per is in miliseconds
%adjust UDP_FC_send_sample_time to larger value (for example 2s)

y = u1;

== matlab function StateFlow_varB/Subsystem6/Subsystem/Subsystem2/Subsystem9/MATLAB Function4 ==
  data: input input; code output; workspace input; pulse_per input
function code = fcn(input, workspace, pulse_per)

coder.extrinsic('set_param')

if input == 1
    code = workspace.Low_servo_open;
else
    code = workspace.Low_servo_close;
end


% if pulse_per == 0
%     if input == 1
%         code = workspace.Low_servo_open;
%     else
%         code = workspace.Low_servo_close;
%     end
% else
%     %comment THIS section if servos are controlled via GSE
%     code = uint8([workspace.FC_ID, workspace.FC_PACKET_LENGTH, workspace.FC_GND_MSG_SERVO_CTRL, workspace.FC_SERVO_IGNORE, workspace.FC_SERVO_PULSE, typecast(uint32(pulse_per), 'uint8'), zeros(1,24)]);
%     set_param('StateFlow_varB/Subsystem6/Constant3', 'Value', '0') %pulse_per is in miliseconds
%     %counting with big endian format
% end

end

== matlab function StateFlow_varB/Subsystem6/Subsystem/Subsystem2/Subsystem9/MATLAB Function3 ==
  data: input input; code output; workspace input
function code = fcn(input, workspace)

if input == 1
    code = workspace.N2O_fill_valve_open;
else
    code = workspace.N2O_fill_valve_close;
end

end

== matlab function StateFlow_varB/Subsystem6/Subsystem/Subsystem2/Subsystem10/MATLAB Function ==
  data: input input; code output; workspace input
function code = fcn(input, workspace)

if input == 1
    code = workspace.N2_fill_valve_open; 
else 
    code = workspace.N2_fill_valve_close; 
end
     
end

== matlab function StateFlow_varB/Subsystem6/Subsystem/Subsystem2/Subsystem10/MATLAB Function1 ==
  data: input input; code output; workspace input
function code = fcn(input, workspace)

if input == 1
    code = workspace.N2_release_valve_open;
else
    code = workspace.N2_release_valve_close;
end
     
end

== matlab function StateFlow_varB/Subsystem6/Subsystem/Subsystem2/Subsystem10/MATLAB Function2 ==
  data: input input; code output; workspace input; pulse_per input
function code = fcn(input, workspace, pulse_per)

coder.extrinsic('set_param')

if input == 1
    code = workspace.High_servo_open;
else
    code = workspace.High_servo_close;
end


% if pulse_per == 0
%     if input == 1
%         code = workspace.High_servo_open;
%     else
%         code = workspace.High_servo_close;
%     end
% else
%     comment THIS section if servos are controlled via GSE
%     code = uint8([workspace.FC_ID, workspace.FC_PACKET_LENGTH, workspace.FC_GND_MSG_SERVO_CTRL, workspace.FC_SERVO_PULSE, workspace.FC_SERVO_IGNORE, typecast(uint32(pulse_per), 'uint8'), zeros(1,24)]);
%     set_param('StateFlow_varB/Subsystem6/Constant2', 'Value', '0') %pulse_per is in miliseconds
%     counting with big endian format
% end

end

== matlab function StateFlow_varB/Subsystem6/Subsystem/Subsystem2/Subsystem10/MATLAB Function3 ==
  data: input input; code output; workspace input
function code = fcn(input, workspace)

if input == 1
    code = workspace.N2O_fill_valve_open;
else
    code = workspace.N2O_fill_valve_close;
end

end

== matlab function StateFlow_varB/Subsystem6/Subsystem/Subsystem2/Subsystem10/MATLAB Function4 ==
  data: input input; code output; workspace input; pulse_per input
function code = fcn(input, workspace, pulse_per)

coder.extrinsic('set_param')

if input == 1
    code = workspace.Low_servo_open;
else
    code = workspace.Low_servo_close;
end


% if pulse_per == 0
%     if input == 1
%         code = workspace.Low_servo_open;
%     else
%         code = workspace.Low_servo_close;
%     end
% else
%     %comment THIS section if servos are controlled via GSE
%     code = uint8([workspace.FC_ID, workspace.FC_PACKET_LENGTH, workspace.FC_GND_MSG_SERVO_CTRL, workspace.FC_SERVO_IGNORE, workspace.FC_SERVO_PULSE, typecast(uint32(pulse_per), 'uint8'), zeros(1,24)]);
%     set_param('StateFlow_varB/Subsystem6/Constant3', 'Value', '0') %pulse_per is in miliseconds
%     %counting with big endian format
% end

end

== matlab function StateFlow_varB/Subsystem6/Subsystem10/MATLAB Function3 ==
  data: input input; code output; workspace input
function code = fcn(input, workspace)

if input == 1
    code = workspace.N2O_fill_valve_open;
else
    code = workspace.N2O_fill_valve_close;
end

end

== matlab function StateFlow_varB/Subsystem6/Subsystem10/MATLAB Function4 ==
  data: input input; code output; workspace input; pulse_per input
function code = fcn(input, workspace, pulse_per)

coder.extrinsic('set_param')

if input == 1
    code = workspace.Low_servo_open;
else
    code = workspace.Low_servo_close;
end


% if pulse_per == 0
%     if input == 1
%         code = workspace.Low_servo_open;
%     else
%         code = workspace.Low_servo_close;
%     end
% else
%     comment THIS section if servos are controlled via GSE
%     code = uint8([workspace.FC_ID, workspace.FC_PACKET_LENGTH, workspace.FC_GND_MSG_SERVO_CTRL, workspace.FC_SERVO_IGNORE, workspace.FC_SERVO_PULSE, typecast(uint32(pulse_per), 'uint8'), zeros(1,24)]);
%     set_param('StateFlow_varB/Subsystem6/Constant3', 'Value', '0') %pulse_per is in miliseconds
%     counting with big endian format
% end

end

== matlab function StateFlow_varB/Subsystem6/Subsystem10/MATLAB Function5 ==
  data: input input; code output; workspace input
function code = fcn(input, workspace)

if input == 1
    code = workspace.N2O_release_valve_open;
else
    code = workspace.N2O_release_valve_close;
end

end

== matlab function StateFlow_varB/Subsystem6/Subsystem1/MATLAB Function ==
  data: input input; code output; workspace input
function code = fcn(input, workspace)

if input == 1
    code = workspace.N2_fill_valve_open; 
else 
    code = workspace.N2_fill_valve_close; 
end
     
end

== matlab function StateFlow_varB/Subsystem6/Subsystem1/MATLAB Function1 ==
  data: input input; code output; workspace input
function code = fcn(input, workspace)

if input == 1
    code = workspace.N2_release_valve_open;
else
    code = workspace.N2_release_valve_close;
end
     
end

== matlab function StateFlow_varB/Subsystem6/Subsystem1/MATLAB Function2 ==
  data: input input; code output; workspace input; pulse_per input
function code = fcn(input, workspace, pulse_per)

coder.extrinsic('set_param')

if input == 1
    code = workspace.High_servo_open;
else
    code = workspace.High_servo_close;
end


% if pulse_per == 0
%     if input == 1
%         code = workspace.High_servo_open;
%     else
%         code = workspace.High_servo_close;
%     end
% else
%     comment THIS section if servos are controlled via GSE
%     code = uint8([workspace.FC_ID, workspace.FC_PACKET_LENGTH, workspace.FC_GND_MSG_SERVO_CTRL, workspace.FC_SERVO_PULSE, workspace.FC_SERVO_IGNORE, typecast(uint32(pulse_per), 'uint8'), zeros(1,24)]);
%     set_param('StateFlow_varB/Subsystem6/Constant2', 'Value', '0') %pulse_per is in miliseconds
%     counting with big endian format
% end

end

== matlab function StateFlow_varB/Subsystem6/Subsystem1/MATLAB Function3 ==
  data: input input; code output; workspace input
function code = fcn(input, workspace)

if input == 1
    code = workspace.N2O_fill_valve_open;
else
    code = workspace.N2O_fill_valve_close;
end

end

== matlab function StateFlow_varB/Subsystem6/Subsystem1/MATLAB Function4 ==
  data: input input; code output; workspace input; pulse_per input
function code = fcn(input, workspace, pulse_per)

coder.extrinsic('set_param')

if input == 1
    code = workspace.Low_servo_open;
else
    code = workspace.Low_servo_close;
end


% if pulse_per == 0
%     if input == 1
%         code = workspace.Low_servo_open;
%     else
%         code = workspace.Low_servo_close;
%     end
% else
%     %comment THIS section if servos are controlled via GSE
%     code = uint8([workspace.FC_ID, workspace.FC_PACKET_LENGTH, workspace.FC_GND_MSG_SERVO_CTRL, workspace.FC_SERVO_IGNORE, workspace.FC_SERVO_PULSE, typecast(uint32(pulse_per), 'uint8'), zeros(1,24)]);
%     set_param('StateFlow_varB/Subsystem6/Constant3', 'Value', '0') %pulse_per is in miliseconds
%     %counting with big endian format
% end

end

== matlab function StateFlow_varB/Subsystem6/Subsystem1/MATLAB Function5 ==
  data: input input; code output; workspace input
function code = fcn(input, workspace)

if input == 1
    code = workspace.N2O_release_valve_open;
else
    code = workspace.N2O_release_valve_close;
end

end

== stateflow chart StateFlow_varB/Subsystem6/Chart ==
  state OFF
    entry:
    OFF_STATE = 1;
    AUTO_STATE = 0;
    MAN_STATE = 0;
  state MAN
    entry:
    OFF_STATE = 0;
    AUTO_STATE = 0;
    MAN_STATE = 1;
  state AUTO
    entry:
    OFF_STATE = 0;
    AUTO_STATE = 1;
    MAN_STATE = 0;
  (default) -> OFF
  MAN -> (junction 18) [order 2] : [CNTRL == 2]
  (junction 18) -> AUTO : [after(3,sec)]
  OFF -> (junction 14) : [CNTRL == 1]
  (junction 14) -> MAN : [after(3,sec)]
  MAN -> OFF [order 1] : [CNTRL == 0]
  AUTO -> MAN [order 2] : [CNTRL == 1]
  AUTO -> OFF [order 1] : [CNTRL == 0]
  data: CNTRL input; AUTO_STATE output; MAN_STATE output; OFF_STATE output
